simulink model "H175_Stage_01_Anode_Cathode"  (R2023a)
settings: Solver=VariableStepAuto  StartTime=0.0  StopTime=500  RelTol=1e-3
values from neighbouring files (symbols this model uses):
  anode_tube_D = 0.01    [All_Properties.mat]    (also in anode_subsystem_parameters.m; environment_parameters.m)
  D = 0.01    [All_Properties.mat]    (also in anode_subsystem_parameters.m)
  densityHydrogen = 0.0899    [All_Properties.mat]    (also in Valve_Init.m; anode_subsystem_parameters.m)
  Fischer_EMTC120K_supplier_mdot_TLU = [33.385172 57.11265182 82.35238332 173.9183787 230.2050798 50.1655574 86.1774137 122.96585 210.0188714 258.8737112 70.20710678 115.3896052 ... (25 elements, 5x5)]    [All_Properties.mat]    (also in cathode_subsystem_parameters.m = [33.385172 50.1655574 70.20710678 87.4902972 105.3161257)
  Fischer_EMTC120K_supplier_pr_TLU = [2.452176848 3.067593046 4.01020547 5.11549365 6.10066015 2.450765612 3.07166407 4.0616557 5.112468546 6.108742034 2.432340262 3.033516574 ... (25 elements, 5x5)]    [All_Properties.mat]    (also in cathode_subsystem_parameters.m = [2.452176848 2.450765612 2.432340262 2.407245766 2.37067916)
  Kv_VL6112 = 0.8    [All_Properties.mat]    (also in anode_subsystem_parameters.m)
  N2_T = [-56.55 -50 -40 -30 -20 -10 -5 -4 -3 -2 -1 0 ... (52 elements, 1x52)]    [All_Properties.mat]    (also in anode_subsystem_parameters.m = [-56.55 -50 -40 -30 -20 -10 -5 -4 -3 -2 -1 0 1 2 3 4 5 10 20; environment_parameters.m = [-56.55, -50:10:-10, -5:1:5, 10:10:350]; stack_model_harness_parameters.m = [-56.55, -50:10:-10, -5:1:5, 10:10:350])
  p_range = 0.005    [All_Properties.mat]    (also in anode_subsystem_parameters.m)
  r_max = 0.2    [All_Properties.mat]    (also in anode_subsystem_parameters.m)
  r_min = 0.0001    [All_Properties.mat]    (also in anode_subsystem_parameters.m)
  responseTimeValve = 0.013    [All_Properties.mat]    (also in anode_subsystem_parameters.m)
undefined symbols (not defined in the file or in its folder): sigbuilder_block
libraries: fl_lib x168, nesl_utility x116, SimscapeFluids_lib x8, slpidlib x5, simulink x1
(part 1 of 8)
settings Model: Creator=adrian.taveras  LastModifiedBy=adrian.taveras
settings SolverCC: MaxConsecutiveMinStep=20  ZeroCrossAlgorithm=Adaptive
settings DataIOCC: Refine=2
settings OptimizationCC: ReuseModelBlockBuffer=off
settings DebuggingCC: IgnoredZcDiagnostic=none
settings SimscapeCC: SimscapeLogType=all

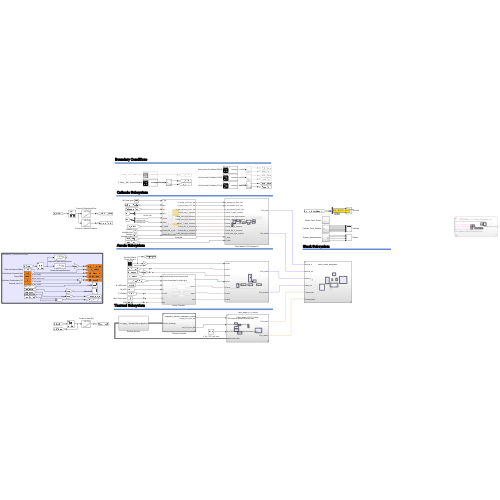
[thumbnail: Simulink's stored preview of the top-level diagram]
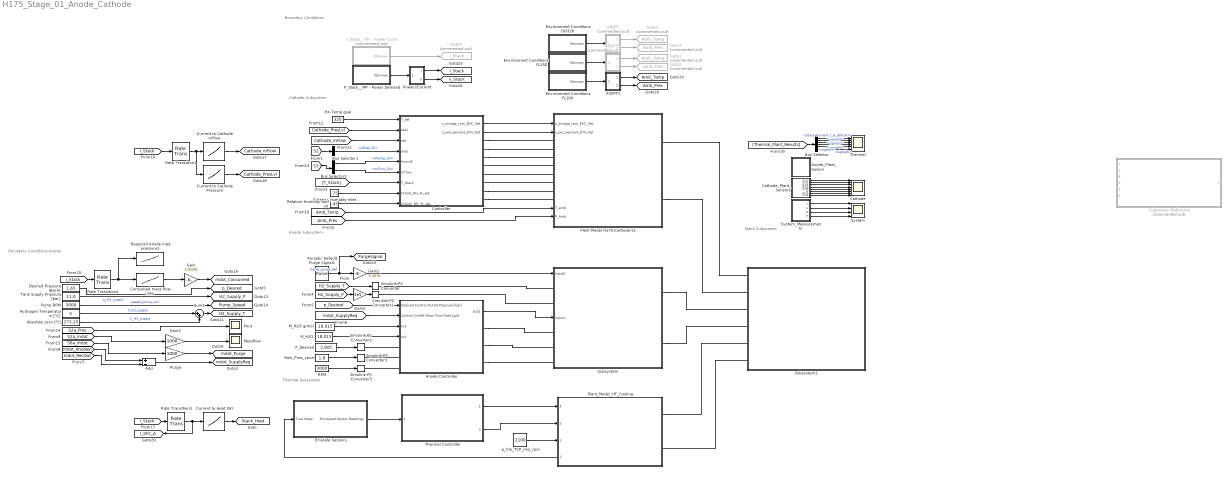
== system H175_Stage_01_Anode_Cathode ==
  note: Anode Subsystem
  note: Boundary Conditions-Anode
  note: Cathode Subsystem
  note: Thermal Subsystem
  note: Stack Subsystem
  note: Boundary Conditions
  "Absolute zero [°C] " : Constant  Value=273.15
  Add : Sum  Inputs=+-
  Alt2PT : Subsystem  Commented=on
  Alt2PT1 : Subsystem  Commented=on
  Alt2PT2 : Subsystem
  Anode Controller : Subsystem
  Anode_Plant_Sensor : Subsystem
  Bus Selector : BusSelector  OutputSignals=Stack Current: I_A_StN (A),signal2,signal3,signal4,signal5,signal6
  Bus Selector1 : BusSelector  OutputSignals=aPres_S2
  Bus Selector2 : BusSelector  OutputSignals=aTemp_S3,mFlow_S3
  Cathode : Scope  NumInputPorts=8
  Cathode_Plant_Sensors : Subsystem
  Consumed mass flow rate : Lookup_n-D  NumberOfTableDimensions=1  BreakpointsForDimension1=[0;20;100;200;300;400;500;600]  Table=[0;0.1;0.5;1;1.5;2;2.5;3]  InternalRulePriority=Speed  RndMeth=Simplest
  Controller : Subsystem
      settings: PortSchema="{\"entries\":[{\"content\":{\"sides\":[{\"content\":{\"connectorIds\":[\"Out1\",\"Out2\",\"LConn1\",\"LConn2\",\"LConn3\",\"LConn4\",\"LConn5\",\"LConn6\",\"LConn7\",\"LConn8\"]},\"type\":\"ConnectorPlacement.EquallySpacedRectSide\",\"uuid\":\"fec6d33c-3ad3-4174-acdc-3a3b9e5715f4\"},{\"content\":{\"connectorIds\":[\"In1\",\"In2\",\"In3\",\"In4\",\"In5\",\"In6\",\"In7\",\"In8\",\"In9\"],\"side\":\"RIGHT\"},\"type\":\"ConnectorPlacement.EquallySpacedRectSide\",\"uuid\":\"4aee90de-c0ab-447d-83f7-53a254285efe\"},{\"content\":{\"side\":\"TOP\"},\"type\":\"ConnectorPlacement.EquallySpacedRectSide\",\"uuid\":\"94b2adb1-5e3a-4413-84ea-fe1e13b8a59d\"}]},\"type\":\"ConnectorPlacement.EquallySpacedConnector\",\"uuid\":\"aca8449a-2e64-4d0b-80a0-10fe30b1ea20\"}],\"packageUris\":[\"http://schema.mathworks.com/mf0/Connector/R2020b\"],\"version\":\"1.0\"}"
  Current to Cathode Pressure : Lookup_n-D  NumberOfTableDimensions=1  BreakpointsForDimension1=[0;50;100;150;200;250;300;350;400;510;600]  Table=[101330;110000;115000;125000;130000;140000;150000;165000;180000;200000;230000]  InternalRulePriority=Speed  RndMeth=Simplest
  Current to Cathode mFlow : Lookup_n-D  NumberOfTableDimensions=1  BreakpointsForDimension1=[0;50;100;150;200;250;300;350;400;510;600]  Table=[0;0.01;0.0225;0.035;0.045;0.055;0.068;0.0825;0.1;0.135;0.167]  InternalRulePriority=Speed  RndMeth=Simplest
  Current to Heat (W) : Lookup_n-D  NumberOfTableDimensions=1  BreakpointsForDimension1=[0:50:400]  Table=[0, 9932, 21438, 33442,47123, 59491, 77033, 93585, 112042]  InternalRulePriority=Speed  RndMeth=Simplest
  Desired Pressure (Bara) : Constant  Value=1.65
  Emulate Sensors : Subsystem
  Environment Conditions DO328 : Subsystem  Tag=STV Subsys  LoadFcn=sigbuilder_block('load');  StartFcn=sigbuilder_block('start');  StopFcn=sigbuilder_block('stop');  ClipboardFcn=sigbuilder_block('clipboard');  mask(Sigbuilder block){tuvar=[0:10]}
      mask help: Simulink:masks:SigbuilderBlock_MD
      mask init:
      | if ~strcmp(get_param(bdroot(gcbh),'SimulationStatus'),'stopped') tuvar = sigbuilder_block('maskInit'); end
      settings: CopyFcn=sigbuilder_block('copy');  DeleteFcn=sigbuilder_block('delete');  ModelCloseFcn=sigbuilder_block('modelClose');  PreSaveFcn=sigbuilder_block('preSave');  PauseFcn=sigbuilder_block('pause');  ContinueFcn=sigbuilder_block('continue');  NameChangeFcn=sigbuilder_block('namechange');  OpenFcn=sigbuilder_block('open',[6 30 1908 951.75 ]);  CloseFcn=sigbuilder_block('close');
      mask Display: plot(0, 0, 100, 100,[2, 2, 32, 32, 2], [68, 8, 8, 68, 68],[32, 2], [38, 38], [32, 19, 2],[53, 60, 44], [32, 17, 17, 2],[16, 16, 31, 31]);txt = getActiveGroup(gcbh);text(2, 100, txt,'verticalAlignment', 'top');
  Environment Conditions FL100 : Subsystem  Tag=STV Subsys  LoadFcn=sigbuilder_block('load');  StartFcn=sigbuilder_block('start');  StopFcn=sigbuilder_block('stop');  ClipboardFcn=sigbuilder_block('clipboard');  mask(Sigbuilder block){tuvar=[0:10]}
      mask help: Simulink:masks:SigbuilderBlock_MD
      mask init:
      | if ~strcmp(get_param(bdroot(gcbh),'SimulationStatus'),'stopped') tuvar = sigbuilder_block('maskInit'); end
      settings: CopyFcn=sigbuilder_block('copy');  DeleteFcn=sigbuilder_block('delete');  ModelCloseFcn=sigbuilder_block('modelClose');  PreSaveFcn=sigbuilder_block('preSave');  PauseFcn=sigbuilder_block('pause');  ContinueFcn=sigbuilder_block('continue');  NameChangeFcn=sigbuilder_block('namechange');  OpenFcn=sigbuilder_block('open',[6 30 1908 951.75 ]);  CloseFcn=sigbuilder_block('close');
      mask Display: plot(0, 0, 100, 100,[2, 2, 32, 32, 2], [68, 8, 8, 68, 68],[32, 2], [38, 38], [32, 19, 2],[53, 60, 44], [32, 17, 17, 2],[16, 16, 31, 31]);txt = getActiveGroup(gcbh);text(2, 100, txt,'verticalAlignment', 'top');
  Environment Conditions FL250 : Subsystem  Tag=STV Subsys  LoadFcn=sigbuilder_block('load');  StartFcn=sigbuilder_block('start');  StopFcn=sigbuilder_block('stop');  ClipboardFcn=sigbuilder_block('clipboard');  mask(Sigbuilder block){tuvar=[0:10]}
      mask help: Simulink:masks:SigbuilderBlock_MD
      mask init:
      | if ~strcmp(get_param(bdroot(gcbh),'SimulationStatus'),'stopped') tuvar = sigbuilder_block('maskInit'); end
      settings: CopyFcn=sigbuilder_block('copy');  DeleteFcn=sigbuilder_block('delete');  ModelCloseFcn=sigbuilder_block('modelClose');  PreSaveFcn=sigbuilder_block('preSave');  PauseFcn=sigbuilder_block('pause');  ContinueFcn=sigbuilder_block('continue');  NameChangeFcn=sigbuilder_block('namechange');  OpenFcn=sigbuilder_block('open',[1920 30 1920 992.25 ]);  CloseFcn=sigbuilder_block('close');
      mask Display: plot(0, 0, 100, 100,[2, 2, 32, 32, 2], [68, 8, 8, 68, 68],[32, 2], [38, 38], [32, 19, 2],[53, 60, 44], [32, 17, 17, 2],[16, 16, 31, 31]);txt = getActiveGroup(gcbh);text(2, 100, txt,'verticalAlignment', 'top');
  Gain : Gain  Gain=1/1000
  Gain1 : Gain  Gain=3.2e-6
  Gain2 : Gain  Gain=1e5
  Gain3 : Gain  Gain=1000
  Goto1 : Goto  Commented=on  GotoTag=Amb_Temp  TagVisibility=global
  Goto2 : Goto  Commented=on  GotoTag=Amb_Pres  TagVisibility=global
  Goto6 : Goto  Commented=on  GotoTag=Amb_Temp  TagVisibility=global
  Goto7 : Goto  Commented=on  GotoTag=Amb_Pres  TagVisibility=global
  Goto9 : Goto  Commented=on  GotoTag=i_Stack  TagVisibility=global
  HX-Temp goal : Constant  Value=320
  Hydrogen Temperature [°C] : Constant  Value=5
  I_Stack__TB -  Power Cycle : Subsystem  Tag=STV Subsys  Commented=on  LoadFcn=sigbuilder_block('load');  StartFcn=sigbuilder_block('start');  StopFcn=sigbuilder_block('stop');  ClipboardFcn=sigbuilder_block('clipboard');  mask(Sigbuilder block){tuvar=[0:10]}
      mask help: Simulink:masks:SigbuilderBlock_MD
      mask init:
      | if ~strcmp(get_param(bdroot(gcbh),'SimulationStatus'),'stopped') tuvar = sigbuilder_block('maskInit'); end
      settings: CopyFcn=sigbuilder_block('copy');  DeleteFcn=sigbuilder_block('delete');  ModelCloseFcn=sigbuilder_block('modelClose');  PreSaveFcn=sigbuilder_block('preSave');  PauseFcn=sigbuilder_block('pause');  ContinueFcn=sigbuilder_block('continue');  NameChangeFcn=sigbuilder_block('namechange');  OpenFcn=sigbuilder_block('open',[161.4 105 550.8 400.2 ]);  CloseFcn=sigbuilder_block('close');
      mask Display: plot(0, 0, 100, 100,[2, 2, 32, 32, 2], [68, 8, 8, 68, 68],[32, 2], [38, 38], [32, 19, 2],[53, 60, 44], [32, 17, 17, 2],[16, 16, 31, 31]);txt = getActiveGroup(gcbh);text(2, 100, txt,'verticalAlignment', 'top');
  M_H2O : Constant  Value=18.015
  M_H2O g/mol : Constant  Value=18.015
  Massflow : Scope
  P_Desired : Constant  Value=2.8e5
  P_Stack__MP - Power Demand : Subsystem  Tag=STV Subsys  LoadFcn=sigbuilder_block('load',[6 30 1908 951.75 ]);  StartFcn=sigbuilder_block('start');  StopFcn=sigbuilder_block('stop');  ClipboardFcn=sigbuilder_block('clipboard');  mask(Sigbuilder block){tuvar=[0:10]}
      mask help: Simulink:masks:SigbuilderBlock_MD
      mask init:
      | if ~strcmp(get_param(bdroot(gcbh),'SimulationStatus'),'stopped') tuvar = sigbuilder_block('maskInit'); end
      settings: CopyFcn=sigbuilder_block('copy');  DeleteFcn=sigbuilder_block('delete');  ModelCloseFcn=sigbuilder_block('modelClose');  PreSaveFcn=sigbuilder_block('preSave');  PauseFcn=sigbuilder_block('pause');  ContinueFcn=sigbuilder_block('continue');  NameChangeFcn=sigbuilder_block('namechange');  OpenFcn=sigbuilder_block('open',[0 30 1920 992.25 ]);  CloseFcn=sigbuilder_block('close');
      mask Display: plot(0, 0, 100, 100,[2, 2, 32, 32, 2], [68, 8, 8, 68, 68],[32, 2], [38, 38], [32, 19, 2],[53, 60, 44], [32, 17, 17, 2],[16, 16, 31, 31]);txt = getActiveGroup(gcbh);text(2, 100, txt,'verticalAlignment', 'top');
  Periodic Default Purge Signal1 : DiscretePulseGenerator  PulseType=Time based  Period=3  PulseWidth=5
  Plant Model H175-Cathode-S1 : Subsystem
      settings: PortSchema="{\"entries\":[{\"content\":{\"sides\":[{\"content\":{\"connectorIds\":[\"In1\",\"In2\",\"LConn1\",\"LConn2\",\"LConn3\",\"LConn4\",\"LConn5\",\"LConn6\",\"LConn7\",\"LConn8\",\"In3\",\"In4\"]},\"type\":\"ConnectorPlacement.EquallySpacedRectSide\",\"uuid\":\"e3b30cb5-20d3-4977-927f-9fea068a9234\"},{\"content\":{\"connectorIds\":[\"RConn1\",\"RConn2\"],\"side\":\"RIGHT\"},\"type\":\"ConnectorPlacement.EquallySpacedRectSide\",\"uuid\":\"2d547627-9665-492a-afa4-fcc16b1173a1\"},{\"content\":{\"side\":\"TOP\"},\"type\":\"ConnectorPlacement.EquallySpacedRectSide\",\"uuid\":\"4ee6a80a-af1f-40b1-aa59-916ec7fe1294\"}]},\"type\":\"ConnectorPlacement.EquallySpacedConnector\",\"uuid\":\"0d82e4d1-cc18-4647-90fc-0df577891cdc\"}],\"packageUris\":[\"http://schema.mathworks.com/mf0/Connector/R2020b\"],\"version\":\"1.0\"}"
  Plant_Model_HT_Cooling : Subsystem  ReferencedSubsystem=Plant_Model_LTHT_Cooling
      settings: PortSchema="{\"entries\":[{\"content\":{\"sides\":[{\"content\":{\"connectorIds\":[\"LConn2\",\"LConn1\"]},\"type\":\"ConnectorPlacement.EquallySpacedRectSide\",\"uuid\":\"706cf171-be05-45fb-992c-ba5e90f5cdb8\"},{\"content\":{\"connectorIds\":[\"Out1\",\"In1\",\"In2\",\"In3\"],\"side\":\"RIGHT\"},\"type\":\"ConnectorPlacement.EquallySpacedRectSide\",\"uuid\":\"bf8ca14f-fef4-4eb5-a927-ccc799898aca\"},{\"content\":{\"side\":\"TOP\"},\"type\":\"ConnectorPlacement.EquallySpacedRectSide\",\"uuid\":\"9ad70fe7-ae85-4ea7-9728-0856e6ff40bf\"}]},\"type\":\"ConnectorPlacement.EquallySpacedConnector\",\"uuid\":\"91c985a6-7405-42c3-ac14-8c35e74d3001\"}],\"packageUris\":[\"http://schema.mathworks.com/mf0/Connector/R2020b\"],\"version\":\"1.0\"}"
  Pout : Scope
  Power2Current : Subsystem
  Pump RPM : Constant  Value=3000
  Purge : Gain  Gain=1000
  RPM : Constant  Value=3000
  Rate Transition1 : RateTransition
  Rate Transition3 : RateTransition
  Rate Transition4 : RateTransition
  Relative Humidity-inlet : Constant  Value=.75
  Relative Humidity-outlet : Constant  Value=.45
  Required Anode Inlet pressure1 : Lookup_n-D  NumberOfTableDimensions=1  BreakpointsForDimension1=[0;20;100;200;300;400;500;600]  Table=[1;1.4;1.6;1.7;1.8;2;2.3;2.6]  InternalRulePriority=Speed  RndMeth=Simplest
  Rezi_Pres_Level : Constant  Value=1.8
  Simulink-PS Converter : nesl_utility/Simulink-PS Converter  PhysicalDomain=network_engine_domain  SubClassName=ps_input  LeftPortType=input  RightPortType=output  PseudoPeriodic=off  Frequencies=[]  NoiseDistribution=none  NoiseParameters=[]  Unit=K  AffineConversion=off  FilteringAndDerivatives=provide  SimscapeFilterOrder=1  InputFilterTimeConstant=0.001  UdotUserProvided=0
  Simulink-PS Converter1 : nesl_utility/Simulink-PS Converter  PhysicalDomain=network_engine_domain  SubClassName=ps_input  LeftPortType=input  RightPortType=output  PseudoPeriodic=off  Frequencies=[]  NoiseDistribution=none  NoiseParameters=[]  Unit=Pa  AffineConversion=off  FilteringAndDerivatives=provide  SimscapeFilterOrder=1  InputFilterTimeConstant=0.001  UdotUserProvided=0
  Simulink-PS Converter2 : nesl_utility/Simulink-PS Converter  PhysicalDomain=network_engine_domain  SubClassName=ps_input  LeftPortType=input  RightPortType=output  PseudoPeriodic=off  Frequencies=[]  NoiseDistribution=none  NoiseParameters=[]  Unit=1  AffineConversion=off  FilteringAndDerivatives=provide  SimscapeFilterOrder=1  InputFilterTimeConstant=0.001  UdotUserProvided=0
  Simulink-PS Converter3 : nesl_utility/Simulink-PS Converter  PhysicalDomain=network_engine_domain  SubClassName=ps_input  LeftPortType=input  RightPortType=output  PseudoPeriodic=off  Frequencies=[]  NoiseDistribution=none  NoiseParameters=[]  Unit=1  AffineConversion=off  FilteringAndDerivatives=provide  SimscapeFilterOrder=1  InputFilterTimeConstant=0.001  UdotUserProvided=0
  Simulink-PS Converter5 : nesl_utility/Simulink-PS Converter  PhysicalDomain=network_engine_domain  SubClassName=ps_input  LeftPortType=input  RightPortType=output  PseudoPeriodic=off  Frequencies=[]  NoiseDistribution=none  NoiseParameters=[]  Unit=1  AffineConversion=off  FilteringAndDerivatives=provide  SimscapeFilterOrder=1  InputFilterTimeConstant=0.001  UdotUserProvided=0
  Subsystem : Subsystem
      settings: PortSchema="{\"entries\":[{\"content\":{\"sides\":[{\"content\":{\"connectorIds\":[\"In1\",\"LConn1\",\"LConn2\",\"In2\",\"LConn3\",\"LConn4\",\"LConn5\"]},\"type\":\"ConnectorPlacement.EquallySpacedRectSide\",\"uuid\":\"6d276737-1cfb-43f0-89a6-ca57f89f04f9\"},{\"content\":{\"connectorIds\":[\"RConn1\",\"RConn2\"],\"side\":\"RIGHT\"},\"type\":\"ConnectorPlacement.EquallySpacedRectSide\",\"uuid\":\"f7ce7b2b-f458-4a7d-a84b-f12d4a9a3d73\"},{\"content\":{\"side\":\"TOP\"},\"type\":\"ConnectorPlacement.EquallySpacedRectSide\",\"uuid\":\"f2759a84-f209-4626-aa5e-b52256180764\"}]},\"type\":\"ConnectorPlacement.EquallySpacedConnector\",\"uuid\":\"a55dce8e-c3c8-40fa-9a6a-dcd78737938e\"}],\"packageUris\":[\"http://schema.mathworks.com/mf0/Connector/R2020b\"],\"version\":\"1.0\"}"
  Subsystem Reference : Subsystem  Commented=on  ReferencedSubsystem=Plant_Model_HT_Cooling_InnerLoop_cryo
      settings: PortSchema="{\"entries\":[{\"content\":{\"sides\":[{\"content\":{\"connectorIds\":[\"In1\",\"In2\",\"In4\",\"In5\",\"In3\",\"In6\",\"LConn1\"]},\"type\":\"ConnectorPlacement.EquallySpacedRectSide\",\"uuid\":\"81f1a8ae-5a2c-41ff-b346-d9b1aace959e\"},{\"content\":{\"connectorIds\":[\"Out1\"],\"side\":\"RIGHT\"},\"type\":\"ConnectorPlacement.EquallySpacedRectSide\",\"uuid\":\"4f9d6f22-7b1b-4528-83d0-ee973e90a06d\"},{\"content\":{\"side\":\"TOP\"},\"type\":\"ConnectorPlacement.EquallySpacedRectSide\",\"uuid\":\"98a2119a-d22a-4110-8b10-12c8af7d6ffc\"}]},\"type\":\"ConnectorPlacement.EquallySpacedConnector\",\"uuid\":\"e3b30cda-fd8e-480b-85c1-c00dafcdf4b3\"}],\"packageUris\":[\"http://schema.mathworks.com/mf0/Connector/R2020b\"],\"version\":\"1.0\"}"
  Subsystem1 : Subsystem  InitFcn=|  ReferencedSubsystem=stack_model_subsystem
      | addpath(genpath('p10_doe_files/'))
      | 
      | addpath('parameters/')
      | run('stack_model_parameters.m')
      | run('physical_constants.m')
      | 
      | addpath('init_scripts/')
      | run('bus_definitions.m')
      settings: PortSchema="{\"entries\":[{\"content\":{\"sides\":[{\"content\":{\"connectorIds\":[\"RConn1\",\"RConn2\",\"LConn1\",\"LConn2\",\"LConn3\",\"LConn4\"]},\"type\":\"ConnectorPlacement.EquallySpacedRectSide\",\"uuid\":\"4512e4dc-d948-48c5-8808-59152d18886b\"},{\"content\":{\"side\":\"RIGHT\"},\"type\":\"ConnectorPlacement.EquallySpacedRectSide\",\"uuid\":\"41925b6c-0186-48b9-82f4-fdd7f73581b7\"},{\"content\":{\"side\":\"TOP\"},\"type\":\"ConnectorPlacement.EquallySpacedRectSide\",\"uuid\":\"9b63b3bb-73f2-49e1-8e7e-b3c18ac9fed6\"}]},\"type\":\"ConnectorPlacement.EquallySpacedConnector\",\"uuid\":\"ec53c91d-995b-4a61-a70a-36f1c25f694d\"}],\"packageUris\":[\"http://schema.mathworks.com/mf0/Connector/R2020b\"],\"version\":\"1.0\"}"
  Sum1 : Sum  Inputs=|++
  System : Scope  NumInputPorts=4
  System_Measurements : Subsystem
  Tank Supply Pressure [bar] : Constant  Value=11.0
  Thermal : Scope  NumInputPorts=6
  Thermal Controller : Subsystem  TreatAsAtomicUnit=on  SystemSampleTime=0.02  ReferencedSubsystem=exemplary_thermal_subsystem_controller
      settings: RTWFcnNameOpts=Use subsystem name  RTWFileNameOpts=Use subsystem name
  p_Vlo_TCP_min_rpm : Constant  Value=2100
  tag scope: Amb_Pres=global, Amb_Temp=global, Cathode_PresLvl=global, Cathode_mFlow=global, H2_Supply_P=global, H2_Supply_T=global, I_SFC_A=global, Pump_Speed=global, PurgeSignal=global, Stack_Heat=global, i_Stack=global, mdot_Consumed=global, mdot_Purge=global, mdot_SupplyReq=global, p_Desired=global, v_Stack=global
  wires:
  Controller/1(s_omega_rpm_EAC_Set) -> Plant Model H175-Cathode-S1/1(s_omega_rpm_EAC_Set)
  Controller/2(s_pos_percent_ETV_Set) -> Plant Model H175-Cathode-S1/2(s_pos_percent_ETV_Set)
  HX-Temp goal/1 -> Controller/1(T_set)
  [Cathode_PresLvl] -> Controller/2(set1)
  [Cathode_mFlow] -> Controller/3(set)
  Bus Selector1/1 -> Controller/4(pres)  "<aPres_S2>"
  Bus Selector2/2 -> Controller/6(mflow)  "<mFlow_S3>"
  Bus Selector2/1 -> Controller/5(humidf)  "<aTemp_S3>"
  [S3] -> Bus Selector2/1
  [Amb_Temp] -> Plant Model H175-Cathode-S1/3(T_amb)
  [Amb_Pres] -> Plant Model H175-Cathode-S1/4(P_Amb)
  Cathode_Plant_Sensors/1(Out1) -> Cathode/1
  Cathode_Plant_Sensors/2(Out2) -> Cathode/2
  Cathode_Plant_Sensors/3(Out3) -> Cathode/3
  Cathode_Plant_Sensors/4(Out4) -> Cathode/4
  Cathode_Plant_Sensors/5(Out5) -> Cathode/5
  Cathode_Plant_Sensors/6(<mFlow_S1>) -> Cathode/6
  Cathode_Plant_Sensors/7(Out7) -> Cathode/7
  Cathode_Plant_Sensors/8(Out8) -> Cathode/8
  [S2] -> Bus Selector1/1
  Relative Humidity-outlet/1 -> Controller/9(CHUwi_RH_%_set)
  Relative Humidity-inlet/1 -> Controller/8(CHUdi_RH_%_set)
  [T_Stack] -> Controller/7(T_Stack)
  Consumed mass flow rate/1 -> Gain/1
  Periodic Default Purge Signal1/1 -> Gain1/1, [PurgeSignal]  "signal_purge_def"
  Anode Controller/1(Out1) -> Subsystem/2(input1)
  Gain3/1 -> Massflow/1
  [S2a_mdot] -> Gain3/1
  [mdot_RecOut] -> Add/2
  M_H2O/1 -> Anode Controller/4(In4)
  Purge/1 -> [mdot_Purge]
  [S6a_mdot] -> Purge/1
  M_H2O g/mol/1 -> Anode Controller/3(In3)
  Rezi_Pres_Level/1 -> Simulink-PS Converter3/1
  Add/1 -> [mdot_SupplyReq]
  [mdot_Anodein] -> Add/1
  [mdot_SupplyReq] -> Anode Controller/2(Control Outlet Mass Flow Rate [g/s])
  Gain/1 -> [mdot_Consumed]
  Gain2/1 -> Simulink-PS Converter1/1
  Hydrogen Temperature [°C]/1 -> Sum1/1  "T_H2_supply"
  [S2a_Pres] -> Pout/1
  [H2_Supply_T] -> Simulink-PS Converter/1
  Sum1/1 -> [H2_Supply_T]
  P_Desired/1 -> Simulink-PS Converter2/1
  "Absolute zero [°C] "/1 -> Sum1/2  "C_H2_supply"
  RPM/1 -> Simulink-PS Converter5/1
  Pump RPM/1 -> [Pump_Speed]  "speed_pump_reci"
  [p_Desired] -> Anode Controller/1(Desired Control Outlet Pressure [bar])
  Tank Supply Pressure [bar]/1 -> [H2_Supply_P]  "p_H2_supply"
  Rate Transition4/1 -> Required Anode Inlet pressure1/1, Consumed mass flow rate/1
  Gain1/1 -> Subsystem/1(input0)
  [H2_Supply_P] -> Gain2/1
  System_Measurements/3(P) -> System/3
  System_Measurements/2(v) -> System/2
  System_Measurements/1(i) -> System/1
  System_Measurements/4(T) -> System/4
  Plant_Model_HT_Cooling/1 -> Emulate Sensors/1(True State)
  Thermal Controller/1 -> Plant_Model_HT_Cooling/3
  Emulate Sensors/1(Emulated Sensor Readings) -> Thermal Controller/1
  p_Vlo_TCP_min_rpm/1 -> Plant_Model_HT_Cooling/1
  Thermal Controller/2 -> Plant_Model_HT_Cooling/2
  Environment Conditions FL100/1(Stairway) -> Alt2PT2/1(In1)
  Alt2PT2/1(Out1) -> [Amb_Temp]
  Alt2PT2/2(Out2) -> [Amb_Pres]
  [i_Stack] -> Rate Transition3/1
  Rate Transition3/1 -> [I_SFC_A], Current to Heat (W)/1
  I_Stack__TB -  Power Cycle/1(Stairway) -> Goto9/1
  Alt2PT1/2(Out2) -> Goto2/1
  Alt2PT1/1(Out1) -> Goto1/1
  Environment Conditions FL250/1(Stairway) -> Alt2PT1/1(In1)
  Alt2PT/1(Out1) -> Goto6/1
  Alt2PT/2(Out2) -> Goto7/1
  Environment Conditions DO328/1(Stairway) -> Alt2PT/1(In1)
  Current to Heat (W)/1 -> [Stack_Heat]
  [i_Stack] -> Rate Transition1/1
  Rate Transition1/1 -> Current to Cathode Pressure/1, Current to Cathode mFlow/1
  Current to Cathode mFlow/1 -> [Cathode_mFlow]
  Current to Cathode Pressure/1 -> [Cathode_PresLvl]
  P_Stack__MP - Power Demand/1(Stairway) -> Power2Current/1(In1)
  Power2Current/2(V) -> [v_Stack]
  Power2Current/1(I) -> [i_Stack]
  [Thermal_Plant_Results] -> Bus Selector/1
  Bus Selector/1 -> Thermal/1  "<Stack Current: I_A_StN (A)>"
  Bus Selector/2 -> Thermal/2  "<signal2>"
  Bus Selector/3 -> Thermal/3  "<signal3>"
  Bus Selector/4 -> Thermal/4  "<signal4>"
  Bus Selector/5 -> Thermal/5  "<signal5>"
  Bus Selector/6 -> Thermal/6  "<signal6>"
  [i_Stack] -> Rate Transition4/1
  Desired Pressure (Bara)/1 -> [p_Desired]
  connections:
  Controller/LConn1 -- Plant Model H175-Cathode-S1/LConn1
  Controller/LConn2 -- Plant Model H175-Cathode-S1/LConn2
  Controller/LConn3 -- Plant Model H175-Cathode-S1/LConn3
  Plant Model H175-Cathode-S1/LConn6 -- Controller/LConn6
  Controller/LConn7 -- Plant Model H175-Cathode-S1/LConn7
  Plant Model H175-Cathode-S1/LConn4 -- Controller/LConn4
  Plant Model H175-Cathode-S1/LConn5 -- Controller/LConn5
  Controller/LConn8 -- Plant Model H175-Cathode-S1/LConn8
  Anode Controller/RConn3 -- Subsystem/LConn5
  Simulink-PS Converter3/RConn1 -- Anode Controller/LConn2
  Anode Controller/LConn3 -- Simulink-PS Converter5/RConn1
  Subsystem/LConn2 -- Simulink-PS Converter1/RConn1
  Anode Controller/LConn1 -- Simulink-PS Converter2/RConn1
  Simulink-PS Converter/RConn1 -- Subsystem/LConn1
  Anode Controller/RConn1 -- Subsystem/LConn3
  Anode Controller/RConn2 -- Subsystem/LConn4
  Plant_Model_HT_Cooling/LConn1 -- Subsystem1/LConn3
  Subsystem1/LConn4 -- Plant_Model_HT_Cooling/LConn2
  Plant Model H175-Cathode-S1/RConn1 -- Subsystem1/RConn1
  Plant Model H175-Cathode-S1/RConn2 -- Subsystem1/RConn2
  Subsystem/RConn1 -- Subsystem1/LConn1
  Subsystem/RConn2 -- Subsystem1/LConn2

== system H175_Stage_01_Anode_Cathode/Alt2PT ==
  In1 : Inport
  Add1 : Sum  Inputs=-+
  Constant4 : Constant  Value=0.0065
  Constant5 : Constant  Value=288.15
  Constant6 : Constant  Value=101330
  Constant7 : Constant  Value=4.256
  Constant8 : Constant  Value=288.15
  Divide1 : Product  Inputs=*/
  Math Function1 : Math  Operator=pow
  Product2 : Product
  Product3 : Product
  Out1 : Outport
  Out2 : Outport  Port=2
  wires:
  Constant5/1 -> Divide1/2
  Constant8/1 -> Add1/2
  In1/1 -> Product2/1
  Add1/1 -> Out1/1, Divide1/1
  Constant4/1 -> Product2/2
  Math Function1/1 -> Product3/1
  Constant7/1 -> Math Function1/2
  Divide1/1 -> Math Function1/1
  Product2/1 -> Add1/1
  Constant6/1 -> Product3/2
  Product3/1 -> Out2/1

== system H175_Stage_01_Anode_Cathode/Alt2PT1 ==
  In1 : Inport
  Add1 : Sum  Inputs=-+
  Constant4 : Constant  Value=0.0065
  Constant5 : Constant  Value=288.15
  Constant6 : Constant  Value=101330
  Constant7 : Constant  Value=4.256
  Constant8 : Constant  Value=288.15
  Divide1 : Product  Inputs=*/
  Math Function1 : Math  Operator=pow
  Product2 : Product
  Product3 : Product
  Out1 : Outport
  Out2 : Outport  Port=2
  wires:
  Product3/1 -> Out2/1
  Constant6/1 -> Product3/2
  Product2/1 -> Add1/1
  Divide1/1 -> Math Function1/1
  Constant7/1 -> Math Function1/2
  Math Function1/1 -> Product3/1
  Constant4/1 -> Product2/2
  Add1/1 -> Divide1/1, Out1/1
  In1/1 -> Product2/1
  Constant8/1 -> Add1/2
  Constant5/1 -> Divide1/2

== system H175_Stage_01_Anode_Cathode/Alt2PT2 ==
  In1 : Inport
  Add1 : Sum  Inputs=-+
  Constant4 : Constant  Value=0.0065
  Constant5 : Constant  Value=288.15
  Constant6 : Constant  Value=101330
  Constant7 : Constant  Value=4.256
  Constant8 : Constant  Value=288.15
  Divide1 : Product  Inputs=*/
  Math Function1 : Math  Operator=pow
  Product2 : Product
  Product3 : Product
  Out1 : Outport
  Out2 : Outport  Port=2
  wires:
  Constant5/1 -> Divide1/2
  Constant8/1 -> Add1/2
  In1/1 -> Product2/1
  Add1/1 -> Out1/1, Divide1/1
  Constant4/1 -> Product2/2
  Math Function1/1 -> Product3/1
  Constant7/1 -> Math Function1/2
  Divide1/1 -> Math Function1/1
  Product2/1 -> Add1/1
  Constant6/1 -> Product3/2
  Product3/1 -> Out2/1

== system H175_Stage_01_Anode_Cathode/Anode Controller ==
  Desired Control Outlet Pressure [bar] : Inport
  Control Outlet Mass Flow Rate [g/s] : Inport  Port=2
  In3 : Inport  Port=3
  In4 : Inport  Port=4
  APRV_VL6112 Valve_Control : Subsystem
  ASVValve_Control : Subsystem
  To Workspace3 : ToWorkspace  VariableName=mdot_Liq  SaveFormat=Structure With Time  SampleTime=-1
  WS6114_Control : Subsystem
  compressor map : Subsystem
  Conn1 : PMIOPort  Side=Right
  output : PMIOPort  Port=2  Side=Right
  Conn3 : PMIOPort  Port=3  Side=Left
  p : PMIOPort  Port=4  Side=Left
  cmd : PMIOPort  Port=5  Side=Right
  rpm : PMIOPort  Port=6  Side=Left
  Out1 : Outport
  wires:
  Control Outlet Mass Flow Rate [g/s]/1 -> APRV_VL6112 Valve_Control/2(Control Outlet Mass Flow Rate [g/s])
  WS6114_Control/1(Out1) -> Out1/1
  Desired Control Outlet Pressure [bar]/1 -> APRV_VL6112 Valve_Control/1(Desired Control Outlet Pressure [bar])
  WS6114_Control/2(Out2) -> To Workspace3/1
  In3/1 -> WS6114_Control/1(In1)
  In4/1 -> WS6114_Control/2(In2)
  connections:
  p/RConn1 -- compressor map/LConn1
  ASVValve_Control/RConn1 -- Conn1/RConn1
  compressor map/RConn1 -- cmd/RConn1
  ASVValve_Control/LConn1 -- Conn3/RConn1
  compressor map/LConn2 -- rpm/RConn1
  APRV_VL6112 Valve_Control/RConn1 -- output/RConn1

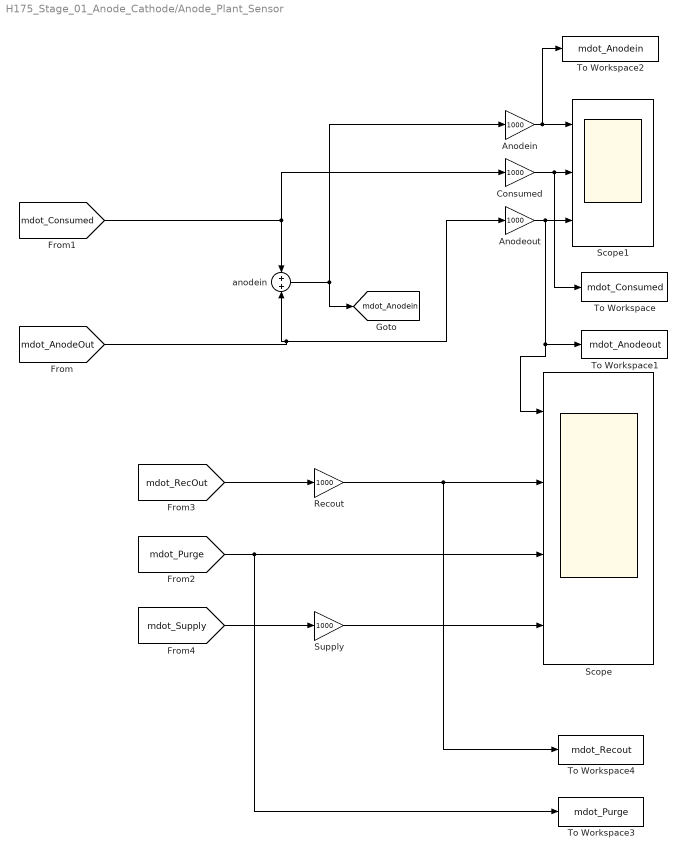
== system H175_Stage_01_Anode_Cathode/Anode_Plant_Sensor ==
  Anodein : Gain  Gain=1000
  Anodeout : Gain  Gain=1000
  Consumed : Gain  Gain=1000
  Recout : Gain  Gain=1000
  Scope : Scope  NumInputPorts=4
  Scope1 : Scope  NumInputPorts=3
  Supply : Gain  Gain=1000
  To Workspace : ToWorkspace  VariableName=mdot_Consumed  SaveFormat=Structure With Time  SampleTime=-1
  To Workspace1 : ToWorkspace  VariableName=mdot_Anodeout  SaveFormat=Structure With Time  SampleTime=-1
  To Workspace2 : ToWorkspace  VariableName=mdot_Anodein  SaveFormat=Structure With Time  SampleTime=-1
  To Workspace3 : ToWorkspace  VariableName=mdot_Purge  SaveFormat=Structure With Time  SampleTime=-1
  To Workspace4 : ToWorkspace  VariableName=mdot_Recout  SaveFormat=Structure With Time  SampleTime=-1
  anodein : Sum
  tag scope: mdot_Anodein=global
  wires:
  [mdot_Consumed] -> anodein/1, Consumed/1
  [mdot_AnodeOut] -> Anodeout/1, anodein/2
  Anodein/1 -> To Workspace2/1, Scope1/1
  Anodeout/1 -> Scope/1, To Workspace1/1, Scope1/3
  Consumed/1 -> To Workspace/1, Scope1/2
  [mdot_Purge] -> To Workspace3/1, Scope/3
  anodein/1 -> [mdot_Anodein], Anodein/1
  Recout/1 -> To Workspace4/1, Scope/2
  [mdot_RecOut] -> Recout/1
  [mdot_Supply] -> Supply/1
  Supply/1 -> Scope/4

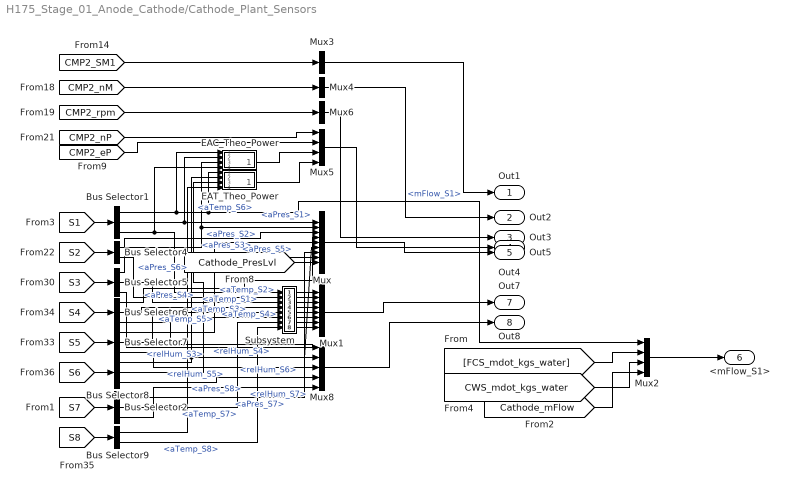
== system H175_Stage_01_Anode_Cathode/Cathode_Plant_Sensors ==
  Bus Selector1 : BusSelector  OutputSignals=mFlow_S1,aPres_S1,aTemp_S1
  Bus Selector2 : BusSelector  OutputSignals=aPres_S7,aTemp_S7,relHum_S7
  Bus Selector4 : BusSelector  OutputSignals=aPres_S2,aTemp_S2
  Bus Selector5 : BusSelector  OutputSignals=aPres_S3,aTemp_S3,relHum_S3
  Bus Selector6 : BusSelector  OutputSignals=aPres_S4,aTemp_S4,relHum_S4
  Bus Selector7 : BusSelector  OutputSignals=aPres_S5,aTemp_S5,relHum_S5
  Bus Selector8 : BusSelector  OutputSignals=aPres_S6,aTemp_S6,relHum_S6
  Bus Selector9 : BusSelector  OutputSignals=aPres_S8,aTemp_S8
  EAC_Theo_Power : Subsystem
  EAT_Theo_Power : Subsystem
  Mux : Mux  Inputs=9
  Mux1 : Mux  Inputs=8
  Mux2 : Mux
  Mux3 : Mux  Inputs=1
  Mux4 : Mux  Inputs=1
  Mux5 : Mux
  Mux6 : Mux  Inputs=1
  Mux8 : Mux  Inputs=5
  Subsystem : Subsystem
  Out1 : Outport
  Out2 : Outport  Port=2
  Out3 : Outport  Port=3
  Out4 : Outport  Port=4
  Out5 : Outport  Port=5
  <mFlow_S1> : Outport  Port=6
  Out7 : Outport  Port=7
  Out8 : Outport  Port=8
  wires:
  [CMP2_eP] -> Mux5/2
  [CMP2_nP] -> Mux5/1
  Mux3/1 -> Out1/1
  [S8] -> Bus Selector9/1
  [CMP2_SM1] -> Mux3/1
  Bus Selector7/3 -> Mux8/3  "<relHum_S5>"
  Bus Selector9/1 -> EAT_Theo_Power/4(<aPres_S7>), Mux/8  "<aPres_S8>"
  Bus Selector4/1 -> EAC_Theo_Power/3(<aPres_S2>), Mux/2  "<aPres_S2>"
  [CMP2_rpm] -> Mux6/1
  [CMP2_nM] -> Mux4/1
  Bus Selector6/1 -> Mux/4  "<aPres_S4>"
  [S5] -> Bus Selector7/1
  Mux/1 -> Out5/1
  Bus Selector5/3 -> Mux8/1  "<relHum_S3>"
  Bus Selector5/1 -> Mux/3  "<aPres_S3>"
  [S4] -> Bus Selector6/1
  Mux6/1 -> Out3/1
  [S3] -> Bus Selector5/1
  Bus Selector1/1 -> Mux2/1, EAT_Theo_Power/1(<mFlow_S1>), EAC_Theo_Power/1(<mFlow_S1>)  "<mFlow_S1>"
  Bus Selector7/1 -> Mux/5  "<aPres_S5>"
  Bus Selector8/1 -> EAT_Theo_Power/2(<aPres_S6>), Mux/6  "<aPres_S6>"
  [S1] -> Bus Selector1/1
  [Cathode_PresLvl] -> Mux/9
  Mux5/1 -> Out4/1
  Bus Selector6/3 -> Mux8/2  "<relHum_S4>"
  Bus Selector8/3 -> Mux8/4  "<relHum_S6>"
  [S6] -> Bus Selector8/1
  Bus Selector1/2 -> Mux/1, EAC_Theo_Power/2(<aPres_S1>)  "<aPres_S1>"
  [S2] -> Bus Selector4/1
  Mux4/1 -> Out2/1
  Mux1/1 -> Out7/1
  Mux8/1 -> Out8/1
  Bus Selector1/3 -> EAC_Theo_Power/4(<aTemp_S1>), Subsystem/1(<aTemp_S1>)  "<aTemp_S1>"
  Bus Selector4/2 -> Subsystem/2(<aTemp_S2>)  "<aTemp_S2>"
  Bus Selector5/2 -> Subsystem/3(<aTemp_S3>)  "<aTemp_S3>"
  Bus Selector6/2 -> Subsystem/4(<aTemp_S4>)  "<aTemp_S4>"
  Bus Selector7/2 -> Subsystem/5(<aTemp_S5>)  "<aTemp_S5>"
  Bus Selector8/2 -> EAT_Theo_Power/3(<aTemp_S6>), Subsystem/6(<aTemp_S6>)  "<aTemp_S6>"
  Bus Selector9/2 -> Subsystem/8(<aTemp_S7>)  "<aTemp_S8>"
  Subsystem/1(Out1) -> Mux1/1
  Subsystem/2(Out2) -> Mux1/2
  Subsystem/3(Out3) -> Mux1/3
  Subsystem/4(Out4) -> Mux1/4
  Subsystem/5(Out5) -> Mux1/5
  Subsystem/6(Out6) -> Mux1/6
  Subsystem/7(Out7) -> Mux1/7
  EAC_Theo_Power/1(Out1) -> Mux5/3
  EAT_Theo_Power/1(Out1) -> Mux5/4
  [S7] -> Bus Selector2/1
  Bus Selector2/2 -> Subsystem/7(In8)  "<aTemp_S7>"
  Subsystem/8(Out8) -> Mux1/8
  Bus Selector2/1 -> Mux/7  "<aPres_S7>"
  Bus Selector2/3 -> Mux8/5  "<relHum_S7>"
  [FCS_mdot_kgs_water] -> Mux2/2
  Mux2/1 -> <mFlow_S1>/1
  [Cathode_mFlow] -> Mux2/4
  [CWS_mdot_kgs_water] -> Mux2/3

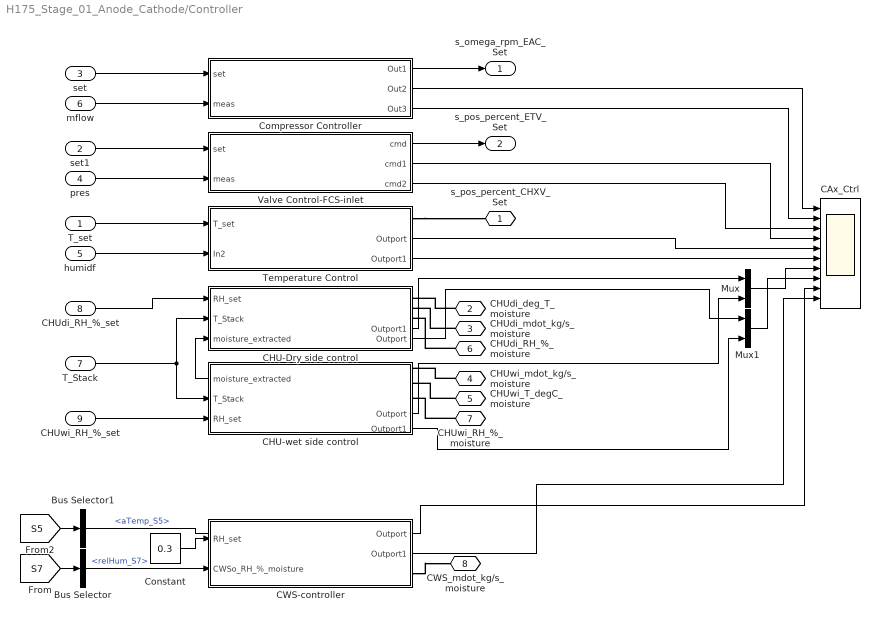
== system H175_Stage_01_Anode_Cathode/Controller ==
  T_set : Inport
  set1 : Inport  Port=2
  set : Inport  Port=3
  pres : Inport  Port=4
  humidf : Inport  Port=5
  mflow : Inport  Port=6
  T_Stack : Inport  Port=7
  CHUdi_RH_%_set : Inport  Port=8
  CHUwi_RH_%_set : Inport  Port=9
  Bus Selector : BusSelector  OutputSignals=relHum_S7
  Bus Selector1 : BusSelector  OutputSignals=aTemp_S5
  CAx_Ctrl : Scope  NumInputPorts=10
  CHU-Dry side control : Subsystem
      settings: PortSchema="{\"entries\":[{\"content\":{\"sides\":[{\"content\":{\"connectorIds\":[\"In1\",\"In2\",\"In3\"]},\"type\":\"ConnectorPlacement.EquallySpacedRectSide\",\"uuid\":\"e04ad6f8-f772-4509-9e44-7e9617907586\"},{\"content\":{\"connectorIds\":[\"RConn1\",\"RConn2\",\"RConn3\",\"Out1\",\"Out2\"],\"side\":\"RIGHT\"},\"type\":\"ConnectorPlacement.EquallySpacedRectSide\",\"uuid\":\"0d864351-c193-45bf-90b1-984eb87a7782\"},{\"content\":{\"side\":\"TOP\"},\"type\":\"ConnectorPlacement.EquallySpacedRectSide\",\"uuid\":\"4c64baeb-8430-45ec-975f-7b4d4952dc8b\"}]},\"type\":\"ConnectorPlacement.EquallySpacedConnector\",\"uuid\":\"5dd74924-e120-426f-b6cd-4773f3c18ed2\"}],\"packageUris\":[\"http://schema.mathworks.com/mf0/Connector/R2020b\"],\"version\":\"1.0\"}"
  CHU-wet side control : Subsystem
      settings: PortSchema="{\"entries\":[{\"content\":{\"sides\":[{\"content\":{\"connectorIds\":[\"Out3\",\"In1\",\"In2\"]},\"type\":\"ConnectorPlacement.EquallySpacedRectSide\",\"uuid\":\"5d784ad6-2694-4818-a8d0-e3f25f29943b\"},{\"content\":{\"connectorIds\":[\"RConn1\",\"RConn2\",\"RConn3\",\"Out1\",\"Out2\"],\"side\":\"RIGHT\"},\"type\":\"ConnectorPlacement.EquallySpacedRectSide\",\"uuid\":\"0f37eddd-db43-448e-bdba-1f3d3b9c7cf9\"},{\"content\":{\"side\":\"TOP\"},\"type\":\"ConnectorPlacement.EquallySpacedRectSide\",\"uuid\":\"2821bd82-ebdd-4ee5-8462-72507a5a1ef1\"}]},\"type\":\"ConnectorPlacement.EquallySpacedConnector\",\"uuid\":\"01309751-94c6-459a-9af4-24f452a07ce7\"}],\"packageUris\":[\"http://schema.mathworks.com/mf0/Connector/R2020b\"],\"version\":\"1.0\"}"
  CWS-controller : Subsystem
  "Compressor Controller " : Subsystem
  Constant : Constant  Value=0.3
  Mux : Mux  Inputs=2
  Mux1 : Mux  Inputs=2
  Temperature Control : Subsystem
      settings: PortSchema="{\"entries\":[{\"content\":{\"sides\":[{\"content\":{\"connectorIds\":[\"In1\",\"In2\"]},\"type\":\"ConnectorPlacement.EquallySpacedRectSide\",\"uuid\":\"e8458165-2262-49de-87f5-2c7bc958bbf7\"},{\"content\":{\"connectorIds\":[\"RConn1\",\"Out1\",\"Out2\"],\"side\":\"RIGHT\"},\"type\":\"ConnectorPlacement.EquallySpacedRectSide\",\"uuid\":\"42ad841b-551f-4f39-a141-2c874d3391ca\"},{\"content\":{\"side\":\"TOP\"},\"type\":\"ConnectorPlacement.EquallySpacedRectSide\",\"uuid\":\"fd6d4917-3fca-4949-93c2-24e90a6fe24c\"}]},\"type\":\"ConnectorPlacement.EquallySpacedConnector\",\"uuid\":\"b641fb00-fee4-4b18-b8cd-d00bddeb3481\"}],\"packageUris\":[\"http://schema.mathworks.com/mf0/Connector/R2020b\"],\"version\":\"1.0\"}"
  Valve Control-FCS-inlet : Subsystem
      settings: PortSchema="{\"entries\":[{\"content\":{\"sides\":[{\"content\":{\"connectorIds\":[\"Out1\",\"Out2\",\"Out3\"]},\"type\":\"ConnectorPlacement.EquallySpacedRectSide\",\"uuid\":\"8b9549d8-0479-4d9d-bb86-2520a85bd308\"},{\"content\":{\"connectorIds\":[\"In1\",\"In2\"],\"side\":\"RIGHT\"},\"type\":\"ConnectorPlacement.EquallySpacedRectSide\",\"uuid\":\"e3096e7f-7009-48fd-960b-05aa908ba84d\"},{\"content\":{\"connectorIds\":[],\"side\":\"TOP\"},\"type\":\"ConnectorPlacement.EquallySpacedRectSide\",\"uuid\":\"4c3fd166-a148-4bd3-b47b-60debcc19f33\"}]},\"type\":\"ConnectorPlacement.EquallySpacedConnector\",\"uuid\":\"0022fa2c-fa81-4715-9695-0e1425952078\"}],\"packageUris\":[\"http://schema.mathworks.com/mf0/Connector/R2020b\"],\"version\":\"1.0\"}"
  s_pos_percent_CHXV_Set : PMIOPort  Side=Left
  CHUdi_deg_T_moisture : PMIOPort  Port=2  Side=Left
  CHUdi_mdot_kg/s_moisture : PMIOPort  Port=3  Side=Left
  CHUwi_mdot_kg/s_moisture : PMIOPort  Port=4  Side=Left
  CHUwi_T_degC_moisture : PMIOPort  Port=5  Side=Left
  CHUdi_RH_%_moisture : PMIOPort  Port=6  Side=Left
  CHUwi_RH_%_moisture : PMIOPort  Port=7  Side=Left
  CWS_mdot_kg/s_moisture : PMIOPort  Port=8  Side=Left
  s_omega_rpm_EAC_Set : Outport
  s_pos_percent_ETV_Set : Outport  Port=2
  wires:
  "Compressor Controller "/1(Out1) -> s_omega_rpm_EAC_Set/1
  humidf/1 -> Temperature Control/2(In2)
  T_set/1 -> Temperature Control/1(T_set)
  Valve Control-FCS-inlet/1(cmd) -> s_pos_percent_ETV_Set/1
  mflow/1 -> "Compressor Controller "/2(meas)
  set/1 -> "Compressor Controller "/1(set)
  set1/1 -> Valve Control-FCS-inlet/1(set)
  pres/1 -> Valve Control-FCS-inlet/2(meas)
  "Compressor Controller "/2(Out2) -> CAx_Ctrl/1
  "Compressor Controller "/3(Out3) -> CAx_Ctrl/2
  Valve Control-FCS-inlet/2(cmd1) -> CAx_Ctrl/4
  Valve Control-FCS-inlet/3(cmd2) -> CAx_Ctrl/3
  CHU-wet side control/3(moisture_extracted) -> CHU-Dry side control/3(moisture_extracted)
  T_Stack/1 -> CHU-Dry side control/2(T_Stack), CHU-wet side control/1(T_Stack)
  CHUdi_RH_%_set/1 -> CHU-Dry side control/1(RH_set)
  CHUwi_RH_%_set/1 -> CHU-wet side control/2(RH_set)
  Bus Selector/1 -> CWS-controller/2(CWSo_RH_%_moisture)  "<relHum_S7>"
  Constant/1 -> CWS-controller/1(RH_set)
  [S7] -> Bus Selector/1
  [S5] -> Bus Selector1/1
  Bus Selector1/1 -> ?  "<aTemp_S5>"
  Temperature Control/1(Outport) -> CAx_Ctrl/5
  Temperature Control/2(Outport1) -> CAx_Ctrl/6
  CHU-Dry side control/1(Outport1) -> Mux/1
  CHU-wet side control/1(Outport) -> Mux/2
  CHU-Dry side control/2(Outport) -> Mux1/1
  CHU-wet side control/2(Outport1) -> Mux1/2
  Mux/1 -> CAx_Ctrl/7
  Mux1/1 -> CAx_Ctrl/8
  CWS-controller/1(Outport) -> CAx_Ctrl/9
  CWS-controller/2(Outport1) -> CAx_Ctrl/10
  connections:
  Temperature Control/RConn1 -- s_pos_percent_CHXV_Set/RConn1
  CHUdi_deg_T_moisture/RConn1 -- CHU-Dry side control/RConn1
  CHUdi_mdot_kg/s_moisture/RConn1 -- CHU-Dry side control/RConn2
  CHUdi_RH_%_moisture/RConn1 -- CHU-Dry side control/RConn3
  CHUwi_mdot_kg/s_moisture/RConn1 -- CHU-wet side control/RConn1
  CHUwi_T_degC_moisture/RConn1 -- CHU-wet side control/RConn2
  CHUwi_RH_%_moisture/RConn1 -- CHU-wet side control/RConn3
  CWS-controller/RConn1 -- CWS_mdot_kg/s_moisture/RConn1

== system H175_Stage_01_Anode_Cathode/Emulate Sensors ==
  True State : Inport
  Band-Limited White Noise : simulink/Sources/Band-Limited White Noise  Cov=[5e-3, 5e-4, 5e-4]  Ts=0.1  seed=[23341]
  Bus Creator : BusCreator  Inputs=3
  Bus Selector : BusSelector  OutputSignals=Stack Current: I_A_StN (A),Stack Inlet Temperature: TSens_CLSti 6812 (°C),Stack Outlet Temperature: TSens_CLSto 6820 (°C)
  Constant : Constant  Value=zeros(1,3)
  Demux : Demux  Outputs=3
  Manual Switch : ManualSwitch  CurrentSetting=0
  Mux : Mux  Inputs=3
  Sum : Sum  Inputs=++|
  Emulated Sensor Readings : Outport
  wires:
  Bus Creator/1 -> Emulated Sensor Readings/1
  True State/1 -> Bus Selector/1
  Bus Selector/1 -> Mux/1  "<Stack Current: I_A_StN (A)>"
  Bus Selector/2 -> Mux/2  "<Stack Inlet Temperature: TSens_CLSti 6812 (°C)>"
  Bus Selector/3 -> Mux/3  "<Stack Outlet Temperature: TSens_CLSto 6820 (°C)>"
  Mux/1 -> Sum/2
  Sum/1 -> Demux/1
  Manual Switch/1 -> Sum/1
  Band-Limited White Noise/1 -> Manual Switch/1  "Signal Noise"
  Constant/1 -> Manual Switch/2
  Demux/1 -> Bus Creator/1  "s_I_A_StN_Get"
  Demux/3 -> Bus Creator/3  "s_T_decC_CLSto_Get"
  Demux/2 -> Bus Creator/2  "s_T_decC_CLSti_Get"

== system H175_Stage_01_Anode_Cathode/Environment Conditions DO328 ==
  Demux : Demux  Tag=STV Demux  Outputs=1
      settings: DisplayOption=none
  FromWs : FromWorkspace  Tag=STV FromWs  VariableName=tuvar
      SigBuilderData=|
      | common.afterFinalStr = 'Extrapolate'
      | common.sampleTime = 0
      | dataSet.timeRange = [0 22226]
      | dataSet.name = 'Group 1'
      | sbobj.Groups.Name = 'Group 1'
      | sbobj.Groups.Signals.Name = 'Stairway'
      | sbobj.Groups.Signals.XData = [0 1 1.1 1.2 1.3 120 270 670 1450 7450 7510 21146 21826 22226]
      | sbobj.Groups.Signals.YData = [0 0 0 0 0 0 1524 4572 8534.4 8534.4 8229.4 8229.6 3048 0]
      | sbobj.Groups.TimeRange = [0 22226]
  Stairway : Outport  Tag=STV Outport
  wires:
  Demux/1 -> Stairway/1
  FromWs/1 -> Demux/1

== system H175_Stage_01_Anode_Cathode/Environment Conditions FL100 ==
  Demux : Demux  Tag=STV Demux  Outputs=1
      settings: DisplayOption=none
  FromWs : FromWorkspace  Tag=STV FromWs  VariableName=tuvar
      SigBuilderData=|
      | common.afterFinalStr = 'Extrapolate'
      | common.sampleTime = 0
      | dataSet.timeRange = [0 22226]
      | dataSet.name = 'Group 1'
      | sbobj.Groups.Name = 'Group 1'
      | sbobj.Groups.Signals.Name = 'Stairway'
      | sbobj.Groups.Signals.XData = [0 1 1.1 1.2 1.3 120 270 670 1450 7450 7510 21146 21826 22226]
      | sbobj.Groups.Signals.YData = [0 0 0 0 0 0 250 650 1100 1100 1000 1000 500 0]
      | sbobj.Groups.TimeRange = [0 22226]
  Stairway : Outport  Tag=STV Outport
  wires:
  Demux/1 -> Stairway/1
  FromWs/1 -> Demux/1

== system H175_Stage_01_Anode_Cathode/Environment Conditions FL250 ==
  Demux : Demux  Tag=STV Demux  Outputs=1
      settings: DisplayOption=none
  FromWs : FromWorkspace  Tag=STV FromWs  VariableName=tuvar
      SigBuilderData=|
      | common.afterFinalStr = 'Extrapolate'
      | common.sampleTime = 0
      | dataSet.timeRange = [0 22226]
      | dataSet.name = 'Group 1'
      | sbobj.Groups.Name = 'Group 1'
      | sbobj.Groups.Signals.Name = 'Stairway'
      | sbobj.Groups.Signals.XData = [0 1 1.1 1.2 1.3 120 320 920 1460 7450 7510 21146 21826 22226]
      | sbobj.Groups.Signals.YData = [0 0 0 0 0 0 1524 4572 7620 7620 7315.2 7315.2 3048 0]
      | sbobj.Groups.TimeRange = [0 22226]
  Stairway : Outport  Tag=STV Outport
  wires:
  FromWs/1 -> Demux/1
  Demux/1 -> Stairway/1

== system H175_Stage_01_Anode_Cathode/I_Stack__TB -  Power Cycle ==
  Demux : Demux  Tag=STV Demux  Outputs=1
      settings: DisplayOption=none
  FromWs : FromWorkspace  Tag=STV FromWs  VariableName=tuvar
      SigBuilderData=|
      | common.afterFinalStr = 'Extrapolate'
      | common.sampleTime = 0
      | dataSet.timeRange = [0 600]
      | dataSet.name = 'Group 1'
      | sbobj.Groups.Name = 'Group 1'
      | sbobj.Groups.Signals.Name = 'Stairway'
      | sbobj.Groups.Signals.XData = [0 180 190 250 260 320 330 390 400 460 470 530 540 600]
      | sbobj.Groups.Signals.YData = [100 100 200 200 300 300 400 400 300 300 200 200 100 100]
      | sbobj.Groups.TimeRange = [0 600]
  Stairway : Outport  Tag=STV Outport
  wires:
  Demux/1 -> Stairway/1
  FromWs/1 -> Demux/1

== system H175_Stage_01_Anode_Cathode/P_Stack__MP - Power Demand ==
  Demux : Demux  Tag=STV Demux  Outputs=1
      settings: DisplayOption=none
  FromWs : FromWorkspace  Tag=STV FromWs  VariableName=tuvar
      SigBuilderData=|
      | common.afterFinalStr = 'Extrapolate'
      | common.sampleTime = 0
      | dataSet.timeRange = [0 22226]
      | dataSet.name = 'Group 1'
      | sbobj.Groups.Name = 'Group 1'
      | sbobj.Groups.Signals.Name = 'Stairway'
      | sbobj.Groups.Signals.XData = [0 1 1.1 1.2 1.3 60 120 5000 5000 21146 21826 22226]
      | sbobj.Groups.Signals.YData = [0 0 0 0 1 1 100 100 85 85 25 1]
      | sbobj.Groups.TimeRange = [0 22226]
  Stairway : Outport  Tag=STV Outport
  wires:
  FromWs/1 -> Demux/1
  Demux/1 -> Stairway/1
